simulink model "EV_Torque_Control"  (R2026a)
settings: Solver=FixedStepDiscrete  StopTime=10  FixedStep=0.01
libraries: simulink x10
settings Model: Creator=ghazal  LastModifiedBy=ghazal

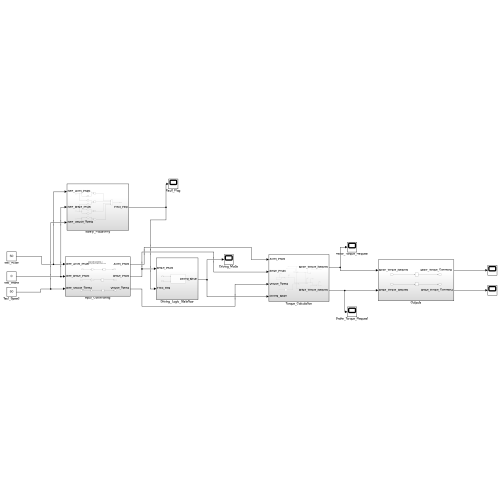
[thumbnail: Simulink's stored preview of the top-level diagram]
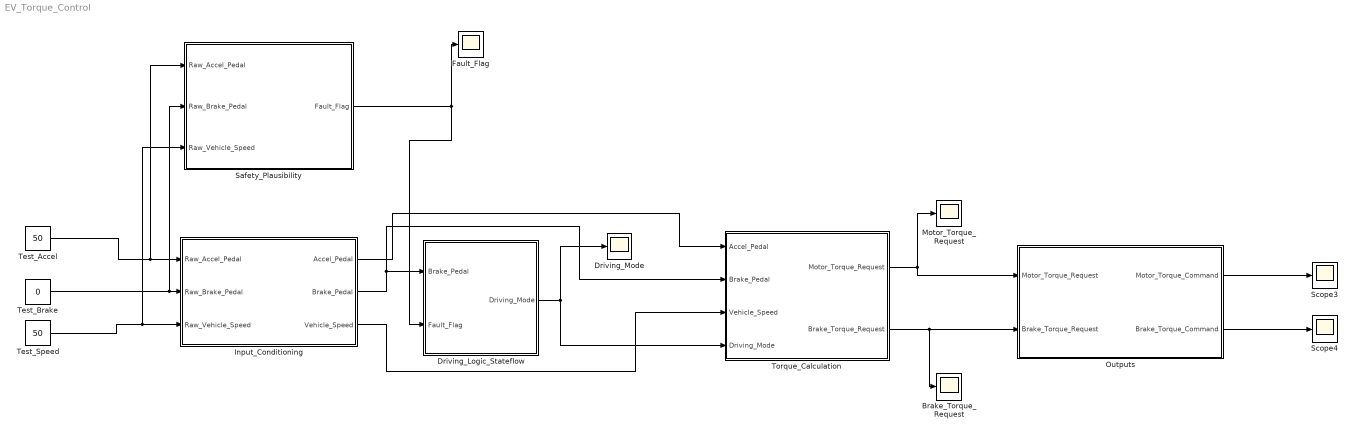
== system EV_Torque_Control ==
  Brake_Torque_Request : Scope
      settings: ActiveDisplayYMinimum=-1  ActiveDisplayYMaximum=1  DataLoggingVariableName=ScopeData2
  Driving_Logic_Stateflow : Subsystem
  Driving_Mode : Scope
      settings: ActiveDisplayYMinimum=-1  ActiveDisplayYMaximum=1
  Fault_Flag : Scope
      settings: ActiveDisplayYMinimum=-1  ActiveDisplayYMaximum=1  DataLoggingVariableName=ScopeData10
  Input_Conditioning : Subsystem
  Motor_Torque_Request : Scope
      settings: ActiveDisplayYMinimum=-1  ActiveDisplayYMaximum=1
  Outputs : Subsystem
  Safety_Plausibility : Subsystem
  Scope3 : Scope
      settings: ActiveDisplayYMinimum=-1  ActiveDisplayYMaximum=1  DataLoggingVariableName=ScopeData11
  Scope4 : Scope
      settings: ActiveDisplayYMinimum=-1  ActiveDisplayYMaximum=1  DataLoggingVariableName=ScopeData12
  Test_Accel : Constant  Value=50
  Test_Brake : Constant  Value=0
  Test_Speed : Constant  Value=50
  Torque_Calculation : Subsystem
  wires:
  Input_Conditioning/1(Accel_Pedal) -> Torque_Calculation/1(Accel_Pedal)
  Input_Conditioning/2(Brake_Pedal) -> Torque_Calculation/2(Brake_Pedal), Driving_Logic_Stateflow/1(Brake_Pedal)
  Input_Conditioning/3(Vehicle_Speed) -> Torque_Calculation/3(Vehicle_Speed)
  Test_Accel/1 -> Input_Conditioning/1(Raw_Accel_Pedal), Safety_Plausibility/1(Raw_Accel_Pedal)
  Test_Brake/1 -> Safety_Plausibility/2(Raw_Brake_Pedal), Input_Conditioning/2(Raw_Brake_Pedal)
  Test_Speed/1 -> Safety_Plausibility/3(Raw_Vehicle_Speed), Input_Conditioning/3(Raw_Vehicle_Speed)
  Driving_Logic_Stateflow/1(Driving_Mode) -> Driving_Mode/1, Torque_Calculation/4(Driving_Mode)
  Torque_Calculation/1(Motor_Torque_Request) -> Motor_Torque_Request/1, Outputs/1("Motor_Torque_Request ")
  Torque_Calculation/2(Brake_Torque_Request) -> Brake_Torque_Request/1, Outputs/2("Brake_Torque_Request ")
  Safety_Plausibility/1(Fault_Flag) -> Driving_Logic_Stateflow/2(Fault_Flag), Fault_Flag/1
  Outputs/1("Motor_Torque_Command ") -> Scope3/1
  Outputs/2(Brake_Torque_Command) -> Scope4/1

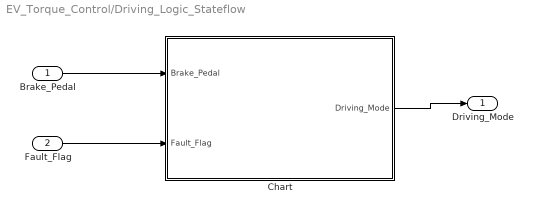
== system EV_Torque_Control/Driving_Logic_Stateflow ==
  Brake_Pedal : Inport
  Fault_Flag : Inport  Port=2
  Chart : Stateflow chart  TreatAsAtomicUnit=on
  Driving_Mode : Outport
  wires:
  Brake_Pedal/1 -> Chart/1(Brake_Pedal)
  Chart/1(Driving_Mode) -> Driving_Mode/1
  Fault_Flag/1 -> Chart/2(Fault_Flag)

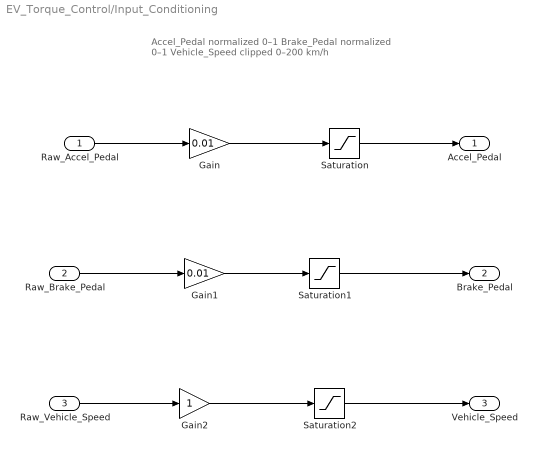
== system EV_Torque_Control/Input_Conditioning ==
  note: Accel_Pedal normalized 0–1
      | Brake_Pedal normalized 0–1
      | Vehicle_Speed clipped 0–200 km/h
  Raw_Accel_Pedal : Inport
  Raw_Brake_Pedal : Inport  Port=2
  Raw_Vehicle_Speed : Inport  Port=3
  Gain : Gain  Gain=0.01
  Gain1 : Gain  Gain=0.01
  Gain2 : Gain
  Saturation : Saturate  UpperLimit=1  LowerLimit=0  LinearizeAsGain=off
  Saturation1 : Saturate  UpperLimit=1  LowerLimit=0  LinearizeAsGain=off
  Saturation2 : Saturate  UpperLimit=200  LowerLimit=0  LinearizeAsGain=off
  Accel_Pedal : Outport
  Brake_Pedal : Outport  Port=2
  Vehicle_Speed : Outport  Port=3
  wires:
  Raw_Accel_Pedal/1 -> Gain/1
  Gain/1 -> Saturation/1
  Saturation/1 -> Accel_Pedal/1
  Raw_Brake_Pedal/1 -> Gain1/1
  Gain1/1 -> Saturation1/1
  Saturation1/1 -> Brake_Pedal/1
  Saturation2/1 -> Vehicle_Speed/1
  Gain2/1 -> Saturation2/1
  Raw_Vehicle_Speed/1 -> Gain2/1

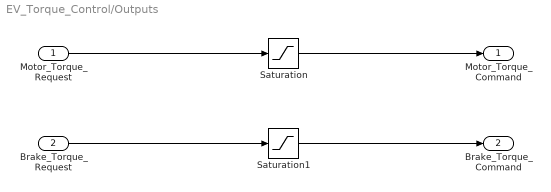
== system EV_Torque_Control/Outputs ==
  "Motor_Torque_Request " : Inport
  "Brake_Torque_Request " : Inport  Port=2
  Saturation : Saturate  UpperLimit=200  LowerLimit=-150
  Saturation1 : Saturate  UpperLimit=300  LowerLimit=0
  "Motor_Torque_Command " : Outport
  Brake_Torque_Command : Outport  Port=2
  wires:
  "Motor_Torque_Request "/1 -> Saturation/1
  Saturation/1 -> "Motor_Torque_Command "/1
  Saturation1/1 -> Brake_Torque_Command/1
  "Brake_Torque_Request "/1 -> Saturation1/1

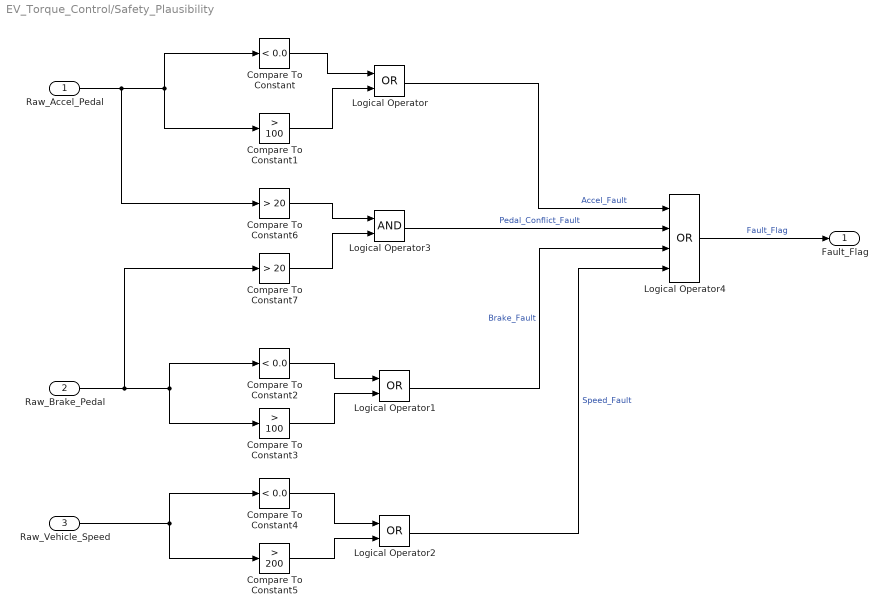
== system EV_Torque_Control/Safety_Plausibility ==
  Raw_Accel_Pedal : Inport
  Raw_Brake_Pedal : Inport  Port=2
  Raw_Vehicle_Speed : Inport  Port=3
  Compare To Constant : simulink/Logic and Bit Operations/Compare To Constant  relop=<  const=0.0  OutDataTypeStr=boolean
  Compare To Constant1 : simulink/Logic and Bit Operations/Compare To Constant  relop=>  const=100  OutDataTypeStr=boolean
  Compare To Constant2 : simulink/Logic and Bit Operations/Compare To Constant  relop=<  const=0.0  OutDataTypeStr=boolean
  Compare To Constant3 : simulink/Logic and Bit Operations/Compare To Constant  relop=>  const=100  OutDataTypeStr=boolean
  Compare To Constant4 : simulink/Logic and Bit Operations/Compare To Constant  relop=<  const=0.0  OutDataTypeStr=boolean
  Compare To Constant5 : simulink/Logic and Bit Operations/Compare To Constant  relop=>  const=200  OutDataTypeStr=boolean
  Compare To Constant6 : simulink/Logic and Bit Operations/Compare To Constant  relop=>  const=20  OutDataTypeStr=boolean
  Compare To Constant7 : simulink/Logic and Bit Operations/Compare To Constant  relop=>  const=20  OutDataTypeStr=boolean
  Logical Operator : Logic  Operator=OR  AllPortsSameDT=off  OutDataTypeStr=boolean
  Logical Operator1 : Logic  Operator=OR  AllPortsSameDT=off  OutDataTypeStr=boolean
  Logical Operator2 : Logic  Operator=OR  AllPortsSameDT=off  OutDataTypeStr=boolean
  Logical Operator3 : Logic  AllPortsSameDT=off  OutDataTypeStr=boolean
  Logical Operator4 : Logic  Operator=OR  Inputs=4  AllPortsSameDT=off  OutDataTypeStr=boolean
  Fault_Flag : Outport
  wires:
  Raw_Accel_Pedal/1 -> Compare To Constant6/1, Compare To Constant/1, Compare To Constant1/1
  Compare To Constant/1 -> Logical Operator/1
  Compare To Constant1/1 -> Logical Operator/2
  Logical Operator/1 -> Logical Operator4/1  "Accel_Fault"
  Raw_Brake_Pedal/1 -> Compare To Constant7/1, Compare To Constant3/1, Compare To Constant2/1
  Compare To Constant2/1 -> Logical Operator1/1
  Compare To Constant3/1 -> Logical Operator1/2
  Logical Operator1/1 -> Logical Operator4/3  "Brake_Fault"
  Raw_Vehicle_Speed/1 -> Compare To Constant4/1, Compare To Constant5/1
  Compare To Constant4/1 -> Logical Operator2/1
  Compare To Constant5/1 -> Logical Operator2/2
  Logical Operator2/1 -> Logical Operator4/4  "Speed_Fault"
  Compare To Constant6/1 -> Logical Operator3/1
  Compare To Constant7/1 -> Logical Operator3/2
  Logical Operator3/1 -> Logical Operator4/2  "Pedal_Conflict_Fault"
  Logical Operator4/1 -> Fault_Flag/1  "Fault_Flag"

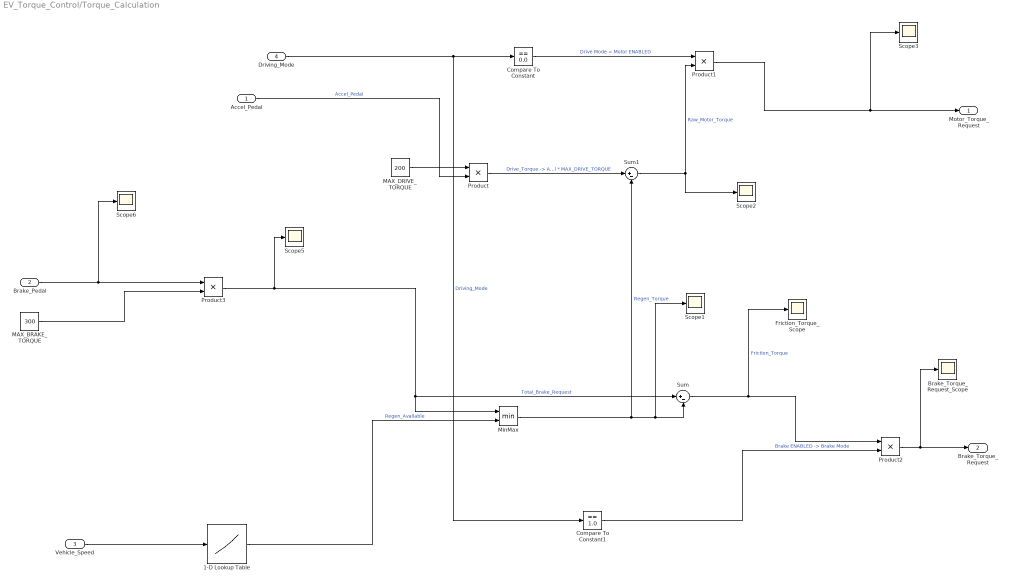
== system EV_Torque_Control/Torque_Calculation ==
  Accel_Pedal : Inport
  Brake_Pedal : Inport  Port=2
  Vehicle_Speed : Inport  Port=3
  Driving_Mode : Inport  Port=4
  1-D Lookup Table : Lookup_n-D  NumberOfTableDimensions=1  BreakpointsForDimension1=[0 5 20 200]  Table=[0 0 150 150]  ExtrapMethod=Clip  InternalRulePriority=Speed  RndMeth=Simplest
  Brake_Torque_Request_Scope : Scope
      settings: ActiveDisplayYMinimum=-99.036438676523488  ActiveDisplayYMaximum=-80.314551010556386  DataLoggingVariableName=ScopeData7
  Compare To Constant : simulink/Logic and Bit Operations/Compare To Constant  relop===  const=0.0  OutDataTypeStr=boolean
  Compare To Constant1 : simulink/Logic and Bit Operations/Compare To Constant  relop===  const=1.0  OutDataTypeStr=boolean
  Friction_Torque_Scope : Scope
      settings: ActiveDisplayYMinimum=20  ActiveDisplayYMaximum=220  DataLoggingVariableName=ScopeData3
  MAX_BRAKE_TORQUE : Constant  Value=300
  MAX_DRIVE_TORQUE : Constant  Value=200
  MinMax : MinMax  Inputs=2
  Product{,1..3} (4 alike) : Product
  Scope{1..3,5..6} (5 alike) : Scope
      Scope1 settings: ActiveDisplayYMinimum=-1  ActiveDisplayYMaximum=1  DataLoggingVariableName=ScopeData4
      Scope2 settings: ActiveDisplayYMinimum=-99.036438676523488  ActiveDisplayYMaximum=-80.314551010556386  DataLoggingVariableName=ScopeData5
      Scope3 settings: ActiveDisplayYMinimum=-99.036438676523488  ActiveDisplayYMaximum=-80.314551010556386  DataLoggingVariableName=ScopeData6
      Scope5 settings: ActiveDisplayYMinimum=-99.036438676523488  ActiveDisplayYMaximum=-80.314551010556386  DataLoggingVariableName=ScopeData8
      Scope6 settings: ActiveDisplayYMinimum=0.19999999999999998  ActiveDisplayYMaximum=0.4  DataLoggingVariableName=ScopeData9
  Sum : Sum  Inputs=|+-
  Sum1 : Sum  Inputs=|+-
  Motor_Torque_Request : Outport
  Brake_Torque_Request : Outport  Port=2
  wires:
  MAX_DRIVE_TORQUE/1 -> Product/1
  Accel_Pedal/1 -> Product/2  "Accel_Pedal"
  Product/1 -> Sum1/1  "Drive_Torque -> Accel_Pedal * MAX_DRIVE_TORQUE"
  Brake_Pedal/1 -> Scope6/1, Product3/1
  MAX_BRAKE_TORQUE/1 -> Product3/2
  Product3/1 -> Scope5/1, Sum/1, MinMax/1  "Total_Brake_Request"
  Vehicle_Speed/1 -> 1-D Lookup Table/1
  1-D Lookup Table/1 -> MinMax/2  "Regen_Available"
  MinMax/1 -> Sum1/2, Scope1/1, Sum/2  "Regen_Torque"
  Sum/1 -> Friction_Torque_Scope/1, Product2/1  "Friction_Torque"
  Sum1/1 -> Product1/2, Scope2/1  "Raw_Motor_Torque"
  Driving_Mode/1 -> Compare To Constant1/1, Compare To Constant/1  "Driving_Mode"
  Compare To Constant/1 -> Product1/1  "Drive Mode = Motor ENABLED"
  Product1/1 -> Scope3/1, Motor_Torque_Request/1
  Compare To Constant1/1 -> Product2/2  "Brake ENABLED -> Brake Mode"
  Product2/1 -> Brake_Torque_Request_Scope/1, Brake_Torque_Request/1

== stateflow chart EV_Torque_Control/Driving_Logic_Stateflow/Chart ==
  state Brake
    entry:
    Driving_Mode = 1;
  state Fault
    entry:
    Driving_Mode = 3;
  state Drive
    entry:
    Driving_Mode = 0;
  Drive -> Brake [order 1] : [Brake_Pedal > 0.01]
  Brake -> Drive [order 1] : [Brake_Pedal <= 0.01]
  Brake -> Fault [order 2] : [Fault_Flag == 1]
  (default) -> Drive
  Drive -> Fault [order 2] : [Fault_Flag == 1]
  data: Brake_Pedal input; Driving_Mode output; Fault_Flag input
